simulink model "Sub4"  (R2024a)
settings: Solver=FixedStepDiscrete  StartTime=0.0  StopTime=4.5  FixedStep=75e-6  RelTol=1e-3  EnableMultiTasking=on
undefined symbols (not defined in the file or in its folder): D1, D11, Delta
libraries: spsSeriesRLCBranchLib x41, spsLoadFlowBusLib x29, spsDistributedParametersLineLib x19, spsThreePhaseSeriesRLCLoadLib x15, spsThreePhaseTransformerTwoWindingsLib x13, spsThreePhaseParallelRLCLoadLib x11, spsThreePhaseVIMeasurementLib x11, spsSynchronousMachinepuStandardLib x7, spsExcitationSystemLib x7, spsHydraulicTurbineandGovernorLib x7, spsGenericPowerSystemStabilizerLib x7, spsMultiBandPowerSystemStabilizerLib x7
(part 1 of 5)
settings Model: Creator=The MathWorks, Inc.  LastModifiedBy=dilu2
settings SolverCC: AlgebraicLoopSolver=TrustRegion
settings DataIOCC: SaveFormat=StructureWithTime  SaveOutput=off  SignalLogging=off  DSMLogging=off  SaveTime=off  ReturnWorkspaceOutputs=off
settings OptimizationCC: ExpressionDepthLimit=2147483647  LifeSpan=inf
settings DebuggingCC: UnderspecifiedInitializationDetection=Classic  MergeDetectMultiDrivingBlocksExec=none  SolverPrmCheckMsg=warning  FcnCallInpInsideContextMsg=warning  UnconnectedInputMsg=warning  UnconnectedOutputMsg=warning  UnconnectedLineMsg=warning  StateNameClashWarn=warning  SFUnexpectedBacktrackingDiag=warning  SFNoUnconditionalDefaultTransitionDiag=warning  SFExecutionAtInitializationDiag=none  ArithmeticOperatorsInVariantConditions=warning
settings HardwareCC: ProdBitPerPointer=32  ProdBitPerSizeT=32  ProdBitPerPtrDiffT=32  ProdLargestAtomicFloat=None  ProdIntDivRoundTo=Undefined  ProdEndianess=Unspecified  ProdWordSize=32  ProdHWDeviceType=32-bit Generic
settings ModelReferenceCC: EnableRefExpFcnMdlSchedulingChecks=on  PropagateSignalLabelsOutOfModel=off
settings SFSimCC: SimUseLocalCustomCode=off  CustomCodeUndefinedFunction=UseInterfaceOnly
settings RTWCC: RTWUseLocalCustomCode=off  GPUComputeCapability=3.5
settings CodeAppCC: StateflowObjectComments=on
settings GRTTargetCC: TargetLangStandard=C89/C90 (ANSI)  CombineOutputUpdateFcns=off  GRTInterface=on
settings ConfigComp: CovMetricSettings=dw  CovSaveCumulativeToWorkspaceVar=on  CovSaveSingleToWorkspaceVar=on  CovExternalEMLEnable=off  CovSFcnEnable=off
settings SimscapeCC: SimscapeNormalizeSystem=off

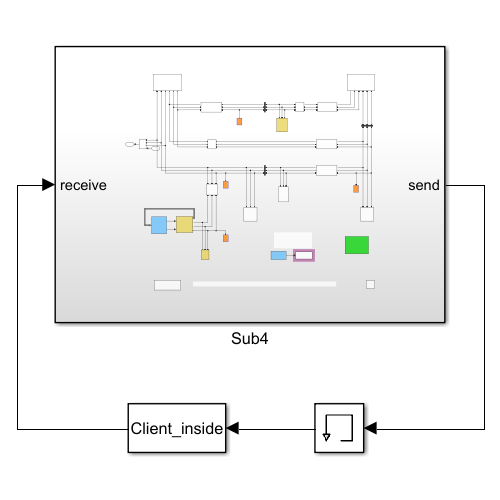
[thumbnail: Simulink's stored preview of the top-level diagram]
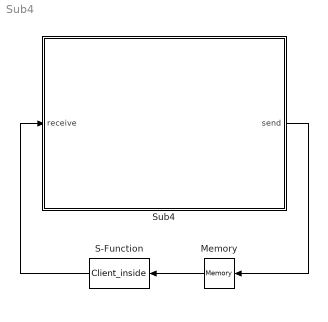
== system Sub4 ==
  Memory : Memory
  S-Function : S-Function  FunctionName=Client_inside  SFunctionDeploymentMode=off  EnableBusSupport=off
  Sub4 : Subsystem
  wires:
  Memory/1 -> S-Function/1
  Sub4/1(send) -> Memory/1
  S-Function/1 -> Sub4/1(receive)

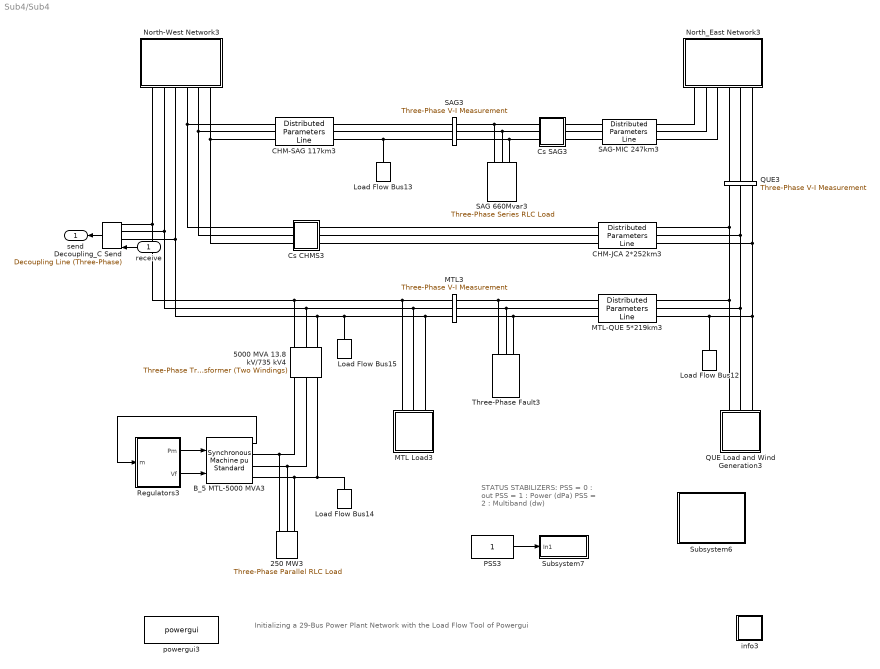
== system Sub4/Sub4 ==
  note: STATUS STABILIZERS:
      | PSS = 0 :  out
      | PSS = 1 :  Power (dPa)
      | PSS = 2 :  Multiband (dw)
  note: Initializing a 29-Bus Power Plant Network with the Load Flow Tool of Powergui
  receive : Inport
  250 MW3 : spsThreePhaseParallelRLCLoadLib/Three-Phase Parallel RLC Load  LConnTagsString=A|B|C  Configuration=Y (grounded)  NominalVoltage=(13800)*1  Vabc=[1e3 1e3 1e3]  Vabcp=[1e3 1e3 1e3]  NominalFrequency=60  UnbalancedPower=off  ActivePower=250000000  InductivePower=0  CapacitivePower=0  Pabc=[10e3 9e3 11e3]  QLabc=[100 90 110]  QCabc=[100 90 110]  Pabcp=[10e3 9e3 11e3]  QLabcp=[100 90 110]  QCabcp=[100 90 110]  Measurements=None  LoadType=constant PQ
  5000 MVA 13.8 kV/735 kV4 : spsThreePhaseTransformerTwoWindingsLib/Three-Phase Transformer (Two Windings)  Winding1Connection=Delta (D1)  Winding2Connection=Yg  CoreType=Three single-phase transformers  SetSaturation=off  Hysteresis=off  DataFile='basic_model'  SetInitialFlux=off  Measurements=None  UNITS=pu  NominalPower=[ 5000e6 60 ]  Winding1="[ 13.8e3 0.002  0.0]"  Winding2=[ 735e3 0.002 0.12]  Rm=500  Lm=500  L0=0.5  Saturation="[ 0,0  ;  0.005,1.2  ;  1.0,1.4 ]"  InitialFluxes=[ 0.8 , -0.8 , 0.7 ]  BreakLoop=off  DiscreteSolver=Trapezoidal iterative  DataType=off  TransfoNumber=0
  B_5 MTL-5000 MVA3 : spsSynchronousMachinepuStandardLib/Synchronous Machine pu Standard  PresetModel=No  MechanicalLoad=Mechanical power Pm  ShowDetailedParameters=on  RotorType=Salient-pole  Units=per unit standard parameters  MeasurementBus=off  NominalParameters="[5000E6  13800   60 ]"  Reactances1=[ 31 32 33 34 35 36 37 ]  Reactances2=[ 1.305, 0.296, 0.252, 0.474, 0.243, 0.18 ]  dAxisTimeConstants=Short-circuit  qAxisTimeConstants=Open-circuit  TimeConstants1=[]  TimeConstants2=[]  TimeConstants3=[]  TimeConstants4=[]  TimeConstants5=[ 1.01, 0.053, 0.1 ]  TimeConstants6=[]  TimeConstants7=[]  TimeConstants8=[]  StatorResistance=2.8544e-3  Mechanical="[ 3.7 0  32]"  PolePairs=32  InitialConditions=[0 -113.876 0.904539 0.904539 0.904539 -42.1129 -162.113 77.8871 1.28555]  SetSaturation=off  Saturation=[0.6404,0.7127,0.8441,0.9214,0.9956,1.082,1.19,1.316,1.457;0.7,0.7698,0.8872,0.9466,0.9969,1.046,1.1,1.151,1.201]  LoadFlowParameters=[1 4000000000 0 0 0]  TsPowergui=0  TsBlock=-1  IterativeModel=Trapezoidal non iterative  IterativeDiscreteModel=Trapezoidal non iterative  BusType=PV  Pref=4500000000  Qref=0  Qmin=-Inf  Qmax=Inf  PLF=0  QLF=0
  CHM-JCA 2*252km3 : spsDistributedParametersLineLib/Distributed Parameters Line  Phases=3  Length=252  Frequency=60  Resistance="[0.01273  0.3864]/2"  Inductance="[0.9337e-3  4.1264e-3]/2"  Capacitance=[12.74e-9 7.751e-9]*2  x1=[-0.0015 2.15568555919851e-08 -52695.4931207272 -817990.56126978;-0.001425 2.15676125923665e-08 -29549.3766895084 -819153.330536763;-0.00135 2.1561128773237e-08 -6379.63893868454 -819661.281164781;-0.001275 2.15374093176625e-08 16795.198597895 -819514.007105874;-0.0012 2.14964731866129e-08 39956.6103096906 -818711.626088671;-0.001125 2.1438353103805e-08 63086.0813185613 -817254.779524281;-0.00105 2.13630955295437e-08 86165.1222792754 -815144.631993557;-0.000975 2.12707606235824e-08 109175.28415961 -812382.870316148;-0.0009 2.11614221970322e-08 132098.172988225 -808971.702202084;-0.000825 2.10351676533583e-08 154915.464558524 -804913.854486961;-0.00075 2.08920979185111e-08 177608.91907674 -800212.570952156;-0.000675 2.07323273602477e-08 200160.395742554 -794871.609731795;-0.0006 2.05559836967078e-08 222551.867250568 -788895.240308557;-0.000525 2.03632078943178e-08 244765.43420106 -782288.240100719;-0.00045 2.01541540551046e-08 266783.339408488 -775055.890643156;-0.000375 1.99289892935087e-08 288587.982096315 -767203.973365366;-0.0003 1.96878936027953e-08 310161.931966798 -758738.764969882;-0.000225 1.94310597111707e-08 331487.943134504 -749667.032414773;-0.00015 1.91586929277182e-08 352548.967912404 -739996.027504242;-7.5e-05 1.88710109782771e-08 373328.170439534 -729733.481091643]  x2=[-0.0015 1.43493457370976e-08 -269861.28631565 -765335.48994974;-0.001425 1.43155296793168e-08 -248116.94439926 -772658.724454069;-0.00135 1.42702700061453e-08 -226174.261593834 -779364.307396144;-0.001275 1.42136028974734e-08 -204050.778544272 -785446.87843556;-0.0012 1.41455736521206e-08 -181764.180424424 -790901.575258095;-0.001125 1.40662366516249e-08 -159332.282799829 -795724.037462569;-0.00105 1.39756553167705e-08 -136773.01738623 -799910.410046481;-0.000975 1.38739020568906e-08 -114104.41771523 -803457.346487641;-0.0009 1.37610582119842e-08 -91344.6047185641 -806362.011419329;-0.000825 1.36372139876944e-08 -68511.7722425057 -808622.082896841;-0.00075 1.35024683831992e-08 -45624.1725039819 -810235.754253618;-0.000675 1.33569291120732e-08 -22700.1015000316 -811201.735545468;-0.0006 1.32007125161829e-08 242.115617734555 -811519.254581725;-0.000525 1.30339434726848e-08 23184.1391919804 -811188.05754253;-0.00045 1.28567552942006e-08 46107.6297200854 -810208.40918173;-0.000375 1.26692896222492e-08 68994.2625144626 -808581.092615234;-0.0003 1.24716963140205e-08 91825.7423510333 -806307.408695007;-0.000225 1.22641333225816e-08 114583.81809415 -803389.174969186;-0.00015 1.20467665706122e-08 137250.297286273 -799828.724229161;-7.5e-05 1.1819769817768e-08 159807.060690745 -795628.902644777]  x3=[-0.0015 5.18178120473788e-11 -353.825063948241 -933.331217283582;-0.001425 5.12281284756022e-11 -327.297425889604 -942.960561677517;-0.00135 5.05974939217388e-11 -300.508151276529 -951.836117826227;-0.001275 4.9926412505402e-11 -273.478655045253 -959.950790745928;-0.0012 4.92154206788081e-11 -246.230544161498 -967.298093691246;-0.001125 4.84650867979448e-11 -218.785600348193 -973.872153340624;-0.00105 4.76760106682359e-11 -191.165762673502 -979.667714491366;-0.000975 4.68488230650662e-11 -163.393110013064 -984.680144260561;-0.0009 4.59841852295494e-11 -135.48984340048 -988.905435788547;-0.000825 4.50827883399416e-11 -107.478268280146 -992.340211441923;-0.00075 4.41453529591247e-11 -79.3807766766213 -994.981725513587;-0.000675 4.31726284585989e-11 -51.2198292947878 -996.827866417607;-0.0006 4.21653924194466e-11 -23.0179375651059 -997.87715837719;-0.000525 4.11244500107463e-11 5.20235435167939 -998.128762604399;-0.00045 4.00506333459326e-11 33.4184875859946 -997.582477970664;-0.000375 3.89448008176175e-11 61.6079065926536 -996.238741167563;-0.0003 3.78078364114041e-11 89.748077181415 -994.098626357737;-0.000225 3.66406489992428e-11 117.816504530469 -991.163844316219;-0.00015 3.54441716128922e-11 145.790751168455 -987.436741062871;-7.5e-05 3.42193606980683e-11 173.648454910629 -982.920295987005]  x4=[-0.0015 3.77673082573545e-11 -3930.11452440301 -10267.8671256384;-0.001425 3.8942548595829e-11 -3638.26562484368 -10374.8700196288;-0.00135 4.00866588567971e-11 -3343.50835141117 -10473.5794012664;-0.001275 4.11987244560214e-11 -3046.07832855995 -10563.9163637817;-0.0012 4.22778564252773e-11 -2746.21331729943 -10645.8086931891;-0.001125 4.33231921229796e-11 -2444.15302513153 -10719.1909260136;-0.00105 4.43338959237659e-11 -2140.13891443214 -10784.0044016209;-0.000975 4.53091598864822e-11 -1834.41400942978 -10840.1973091104;-0.0009 4.62482044000385e-11 -1527.22270193575 -10887.7247287315;-0.000825 4.71502788066187e-11 -1218.81055598109 -10926.5486677923;-0.00075 4.80146620017444e-11 -909.424111516405 -10956.6380910298;-0.000675 4.88406630107148e-11 -599.310687331626 -10977.9689454196;-0.0006 4.96276215409617e-11 -288.718183353157 -10990.5241794029;-0.000525 5.03749085098768e-11 22.1051175235489 -10994.2937565179;-0.00045 5.10819265476911e-11 332.910747907526 -10989.2746634223;-0.000375 5.17481104750028e-11 643.450254533331 -10975.4709123022;-0.0003 5.23729277545734e-11 953.475396870781 -10952.8935376652;-0.000225 5.29558789170297e-11 1262.73834556463 -10921.5605875191;-0.00015 5.34964979601319e-11 1570.99188054559 -10881.4971089448;-7.5e-05 5.39943527212886e-11 1877.98958865422 -10832.7351280741]  x5=0.00142516474882927  V1=ones(3,3)  V2=ones(3,3)  I1=ones(3,3)  I2=ones(3,3)  nHarmo=1  Measurements=None  Decoupling=on  VsMag0=[669271.096488305 669270.65292639 669270.90062483]  VrMag0=[662602.894278686 662603.037872394 662602.72616328]  VsAngle0=[-1.28592943402312 -121.285926872015 118.714104732565]  VrAngle0=[-17.0228975012844 -137.022921456005 102.977079768211]  IsMag0=[819.83811546345 819.831333521039 819.822841412307]  IrMag0=[9030.15416595172 9030.15837069535 9030.16606874901]  IsAngle0=[-18.3607604375278 -138.361719384148 101.639170566751]  IrAngle0=[-18.5448447465977 -138.544772943744 101.455168050312]
      settings: AttributesFormatString=\n  LibrarySourceBlock=sps_lib/Power Grid Elements/Distributed Parameters Line
  CHM-SAG 117km3 : spsDistributedParametersLineLib/Distributed Parameters Line  Phases=3  Length=117  Frequency=60  Resistance="[0.01273  0.3864]"  Inductance="[0.9337e-3  4.1264e-3]"  Capacitance=[12.74e-9 7.751e-9]  x1=[-0.000675 1.98878227916596e-08 120099.384212521 -820048.654169228;-0.0006 1.97251603608904e-08 143234.62761709 -816325.600271039;-0.000525 1.95467299387338e-08 166255.371451905 -811949.988178193;-0.00045 1.93526741597392e-08 189143.213286574 -806925.31568805;-0.000375 1.91431481491271e-08 211879.85693053 -801255.599446916;-0.0003 1.89183193987846e-08 234447.127058726 -794945.371739206;-0.000225 1.86783676333747e-08 256826.983740713 -787999.676864401;-0.00015 1.84234846666673e-08 279001.536861482 -780424.067104709;-7.5e-05 1.81538742482061e-08 300953.060422551 -772224.598286662]  x2=[-0.000675 1.36683940617169e-08 166130.546631601 -803426.098272919;-0.0006 1.35304963284223e-08 188777.466023317 -798408.377649397;-0.000525 1.33817825233862e-08 211273.479597086 -792752.421584839;-0.00045 1.32223715261491e-08 233600.604383858 -786462.751363985;-0.000375 1.3052390767423e-08 255740.992421694 -779544.394852975;-0.0003 1.28719761272257e-08 277676.945023157 -772002.882480148;-0.000225 1.26812718262602e-08 299390.926923368 -763844.242815107;-0.00015 1.24804303106267e-08 320865.580297431 -755074.997749568;-7.5e-05 1.22696121299599e-08 342083.738636013 -745702.157283863]  x3=[-0.000675 1.44875953449933e-11 655.342290943933 -4153.32595111588;-0.0006 1.34518116377455e-11 772.497655199718 -4133.13889809608;-0.000525 1.24052747580941e-11 889.035496649547 -4109.64787708029;-0.00045 1.13488212916082e-11 1004.86265672605 -4082.87166643128;-0.000375 1.02832957510245e-11 1119.88654496969 -4052.83167064216;-0.0003 9.20954990115717e-12 1234.01521304411 -4019.55190322593;-0.000225 8.12844207800969e-12 1347.15742823829 -3983.05896751947;-0.00015 7.04083650263438e-12 1459.22274639654 -3943.38203541722;-7.5e-05 5.94760259028728e-12 1570.12158421818 -3900.55282405163]  x4=[-0.000675 2.92966755964294e-11 -58.1790322608717 -1899.19040567978;-0.0006 2.9950337942892e-11 -4.46495442944831 -1900.07615984023;-0.000525 3.05800584474585e-11 49.2526926182299 -1899.44302219064;-0.00045 3.11853337211928e-11 102.930967817021 -1897.29149885157;-0.000375 3.17656799163019e-11 156.526961575035 -1893.62330971785;-0.0003 3.23206331129171e-11 209.997830074909 -1888.44138708375;-0.000225 3.28497496899441e-11 263.300829522496 -1881.74987329894;-0.00015 3.3352606679687e-11 316.3933503156 -1873.55411745715;-7.5e-05 3.38288021059622e-11 369.232951105443 -1863.86067112021]  x5=0.000661683633385019  V1=ones(3,3)  V2=ones(3,3)  I1=ones(3,3)  I2=ones(3,3)  nHarmo=1  Measurements=None  Decoupling=on  VsMag0=[676709.77841627 676709.532429382 676709.555770597]  VrMag0=[669872.175479969 669872.308250225 669872.011404685]  VsAngle0=[-7.08802978837131 -127.088039531018 112.911983377249]  VrAngle0=[-3.73716141990682 -123.737184181172 116.262817364735]  IsMag0=[3442.59994794247 3442.59576511424 3442.58917191287]  IrMag0=[1555.67453781757 1555.67655932623 1555.68353522262]  IsAngle0=[-6.45330477220923 -126.453471672163 113.546672066868]  IrAngle0=[-17.1748303043271 -137.174490649351 102.825275045855]
      settings: AttributesFormatString=\n  LibrarySourceBlock=sps_lib/Power Grid Elements/Distributed Parameters Line
  Cs CHMS3 : Subsystem  mask{Xc=33/2}
      mask prompts: Xc "Condensator Reactance at  60Hz  (ohm):"
      mask help: Series Compensation
      mask init:
      | Cs=1/Xc/(2*pi*60);
      mask Display: disp('Cs')
  Cs SAG3 : Subsystem  mask{Xc=22}
      mask prompts: Xc "Condensator Reactance at  60Hz  (ohm):"
      mask help: Series Compensation
      mask init:
      | Cs=1/Xc/(2*pi*60);
      mask Display: disp('Cs')
  Decoupling_C Send : spsDecouplingLineThreePhaseLib/Decoupling Line (Three-Phase)  Length=252  Frequency=60  Resistance="[0.01273  0.3864]/2"  Inductance="[0.9337e-3  4.1264e-3]/2"  Capacitance=[12.74e-9 7.751e-9]*2  VsMag0=[645716.873803142 645717.117585011 645717.103800405]  VsAngle0=[95.8608940156725 -144.139117060791 -24.1390927893464]  IhsMag0=[6636.13895490986 6636.14647589719 6636.142035682]  IhsAngle0=[111.871942870307 -128.128050353134 -8.12799750567101]  ShowPorts=on  ConnectorID=T42_4044_2849153755848_S
      settings: LibrarySourceBlock=|
      | sps_lib/Power Grid Elements/Decoupling Line
      | (Three-Phase)
  Load Flow Bus12 : spsLoadFlowBusLib/Load Flow Bus  LConnTagsString=a  Phases=single  Connectors=on one side  ID=QUE7  Vbase=735e3  Vref=1  Vangle=0  VLF=1.023  VLFb=1  VLFc=1  angleLF=-14.99  angleLFb=0  angleLFc=0
      settings: AttributesFormatString=%<ID>\n%<Vbase>V\n%<VLF>pu\n%<angleLF>deg.
  Load Flow Bus13 : spsLoadFlowBusLib/Load Flow Bus  LConnTagsString=a  Phases=single  Connectors=on one side  ID=SAG7  Vbase=735e3  Vref=1  Vangle=0  VLF=1.036  VLFb=1  VLFc=1  angleLF=-0.1653  angleLFb=0  angleLFc=0
      settings: AttributesFormatString=%<ID>\n%<Vbase>V\n%<VLF>pu\n%<angleLF>deg.
  Load Flow Bus14 : spsLoadFlowBusLib/Load Flow Bus  LConnTagsString=a  Phases=single  Connectors=on one side  ID=MTL_13.8  Vbase=13.8e3  Vref=1  Vangle=0  VLF=1  VLFb=1  VLFc=1  angleLF=-47.86  angleLFb=0  angleLFc=0
      settings: AttributesFormatString=%<ID>\n%<Vbase>V\n%<VLF>pu\n%<angleLF>deg.
  Load Flow Bus15 : spsLoadFlowBusLib/Load Flow Bus  LConnTagsString=a  Phases=single  Connectors=on one side  ID=MTL7  Vbase=735e3  Vref=1  Vangle=0  VLF=1.013  VLFb=1  VLFc=1  angleLF=-23.64  angleLFb=0  angleLFc=0
      settings: AttributesFormatString=%<ID>\n%<Vbase>V\n%<VLF>pu\n%<angleLF>deg.
  MTL Load3 : Subsystem
  MTL-QUE 5*219km3 : spsDistributedParametersLineLib/Distributed Parameters Line  Phases=3  Length=219  Frequency=60  Resistance="[0.01273  0.3864]/5"  Inductance="[0.9337e-3  4.1264e-3]/5"  Capacitance=[12.74e-9 7.751e-9]*5  x1=[-0.001275 8.97990123474719e-08 0 0;-0.0012 8.97669453653995e-08 0 0;-0.001125 8.96631200606823e-08 0 0;-0.00105 8.94876194296804e-08 0 0;-0.000975 8.92405837649128e-08 0 0;-0.0009 8.89222105429104e-08 0 0;-0.000825 8.85327542663553e-08 -163872.45963864 -773673.870997357;-0.00075 8.80725262606363e-08 -141934.751428743 -777997.405054978;-0.000675 8.75418944249794e-08 -119883.582750228 -781699.019890759;-0.0006 8.69412829383551e-08 -97736.5809699434 -784775.756490434;-0.000525 8.62711719203961e-08 -75511.450062251 -787225.155357843;-0.00045 8.55320970475971e-08 -53225.9564567427 -789045.258481008;-0.000375 8.47246491251032e-08 -30897.9148360274 -790234.61089734;-0.0003 8.38494736144293e-08 -8545.1738949461 -790792.261856716;-0.000225 8.2907270117488e-08 13814.3979274013 -790717.76558149;-0.00015 8.18987918173386e-08 36162.9267314129 -790011.181622847;-7.5e-05 8.08248448761039e-08 58482.5474451067 -788673.074813191]  x2=[-0.001275 1.42136028974734e-08 0 0;-0.0012 1.41455736521206e-08 0 0;-0.001125 1.40662366516249e-08 0 0;-0.00105 1.39756553167705e-08 0 0;-0.000975 1.38739020568906e-08 0 0;-0.0009 1.37610582119842e-08 0 0;-0.000825 1.36372139876944e-08 -68511.7722425057 -808622.082896841;-0.00075 1.35024683831992e-08 -45624.1725039819 -810235.754253618;-0.000675 1.33569291120732e-08 -22700.1015000316 -811201.735545468;-0.0006 1.32007125161829e-08 242.115617734555 -811519.254581725;-0.000525 1.30339434726848e-08 23184.1391919804 -811188.05754253;-0.00045 1.28567552942006e-08 46107.6297200854 -810208.40918173;-0.000375 1.26692896222492e-08 68994.2625144626 -808581.092615234;-0.0003 1.24716963140205e-08 91825.7423510333 -806307.408695007;-0.000225 1.22641333225816e-08 114583.81809415 -803389.174969186;-0.00015 1.20467665706122e-08 137250.297286273 -799828.724229161;-7.5e-05 1.1819769817768e-08 159807.060690745 -795628.902644777]  x3=[-0.001275 3.56612733394778e-10 0 0;-0.0012 3.31049358806165e-10 0 0;-0.001125 3.05221348425347e-10 0 0;-0.00105 2.79149348768642e-10 0 0;-0.000975 2.52854201393659e-10 0 0;-0.0009 2.26356926238881e-10 0 0;-0.000825 1.99678704820645e-10 -7102.47823834737 -20057.5471743822;-0.00075 1.72840863300962e-10 -6532.60058481158 -20250.3213202489;-0.000675 1.4586485543971e-10 -5957.50087032043 -20426.9076690924;-0.0006 1.18772245444827e-10 -5377.63882078636 -20587.1650604875;-0.000525 9.15846907342113e-11 -4793.4779690596 -20730.9653871275;-0.00045 6.43239246231154e-11 -4205.48528438703 -20858.1936972313;-0.000375 3.70117389508649e-11 -3614.13079912422 -20968.7482864347;-0.0003 9.66996666079572e-12 -3019.88723299863 -21062.5407790905;-0.000225 -1.76795356526667e-11 -2423.22961522482 -21139.4961989151;-0.00015 -4.50149052158343e-11 -1824.63490477324 -21199.5530289235;-7.5e-05 -7.23142905525236e-11 -1224.58160909665 -21242.6632606046]  x4=[-0.001275 2.96404447143572e-10 0 0;-0.0012 3.25528984273917e-10 0 0;-0.001125 3.54393298514994e-10 0 0;-0.00105 3.82974316175637e-10 0 0;-0.000975 4.11249190027634e-10 0 0;-0.0009 4.39195317569445e-10 0 0;-0.000825 4.66790359094306e-10 -1323.85659522578 -8328.03394763841;-0.00075 4.94012255548238e-10 -1087.88942341657 -8362.1315609207;-0.000675 5.20839246163726e-10 -851.052609447551 -8389.5446141781;-0.0006 5.47249885854939e-10 -613.535477044081 -8410.25119383526;-0.000525 5.73223062360603e-10 -375.52789376767 -8424.23474736923;-0.00045 5.98738013120823e-10 -137.22011923875 -8431.48409654126;-0.000375 6.23774341874353e-10 101.197346953951 -8431.99344633255;-0.0003 6.48312034963056e-10 339.533917535869 -8425.76238957667;-0.000225 6.72331477330517e-10 577.599069899151 -8412.79590728505;-0.00015 6.95813468202016e-10 815.202498403518 -8393.10436466524;-7.5e-05 7.18739236433337e-10 1052.15426650368 -8366.70350283512]  x5=0.00123853603172068  V1=ones(3,3)  V2=ones(3,3)  I1=ones(3,3)  I2=ones(3,3)  nHarmo=1  Measurements=None  Decoupling=on  VsMag0=[645717.103800436 645717.117585008 645716.873803144]  VrMag0=[662602.894278686 662603.037872394 662602.72616328]  VsAngle0=[-24.139092789334 -144.139117060794 95.8608940156766]  VrAngle0=[-17.0228975012844 -137.022921456005 102.977079768211]  IsMag0=[17463.0562889063 17463.0593352231 17463.0444100092]  IrMag0=[6920.72764335847 6920.7290374947 6920.73301494311]  IsAngle0=[-31.6792680234199 -151.679318797617 88.3206979336619]  IrAngle0=[-21.2124174849684 -141.212372798418 98.7875948627529]
      settings: AttributesFormatString=\n  LibrarySourceBlock=sps_lib/Power Grid Elements/Distributed Parameters Line
  MTL3 : spsThreePhaseVIMeasurementLib/Three-Phase V-I Measurement  VoltageMeasurement=phase-to-ground  SetLabelV=on  LabelV=Vabc_MTL7_4  Vpu=on  VpuLL=off  CurrentMeasurement=no  SetLabelI=off  LabelI=A1  Ipu=off  Pbase=100e6  Vbase=735e3  OutputType=Magnitude  PhasorSimulation=off  PSBequivalent=0
  North-West Network3 : Subsystem
  North_East Network3 : Subsystem
  PSS3 : Constant
  QUE Load and Wind Generation3 : Subsystem
  QUE3 : spsThreePhaseVIMeasurementLib/Three-Phase V-I Measurement  VoltageMeasurement=no  SetLabelV=on  LabelV=Vabc_QUE7  Vpu=on  VpuLL=off  CurrentMeasurement=no  SetLabelI=off  LabelI=A1  Ipu=off  Pbase=100e6  Vbase=735e3  OutputType=Magnitude  PhasorSimulation=off  PSBequivalent=0
  Regulators3 : Subsystem
  SAG 660Mvar3 : spsThreePhaseSeriesRLCLoadLib/Three-Phase Series RLC Load  LConnTagsString=A|B|C  Configuration=Y (grounded)  NominalVoltage=735e3  Vabc=[1e3 1e3 1e3]  Vabcp=[1e3 1e3 1e3]  NominalFrequency=60  UnbalancedPower=off  ActivePower=2200000  InductivePower=660e6  CapacitivePower=0  Pabc=[10e3 9e3 11e3]  QLabc=[100 90 110]  QCabc=[100 90 110]  Pabcp=[10e3 9e3 11e3]  QLabcp=[100 90 110]  QCabcp=[100 90 110]  Measurements=None  LoadType=constant Z
  SAG-MIC 247km3 : spsDistributedParametersLineLib/Distributed Parameters Line  Phases=3  Length=247  Frequency=60  Resistance="[0.01273  0.3864]/1"  Inductance="[0.9337e-3  4.1264e-3]/1"  Capacitance=[12.74e-9 7.751e-9]*1  x1=[-0.001425 1.51518681270064e-08 -89449.2345901318 -803563.355727012;-0.00135 1.51308920077656e-08 -66696.2840152404 -805770.95443022;-0.001275 1.50978204849643e-08 -43890.0174513944 -807334.432161166;-0.0012 1.50526799954717e-08 -21048.6658791376 -808252.539099673;-0.001125 1.49955066239044e-08 1809.51167456759 -808524.541325103;-0.00105 1.49263460737809e-08 24666.2427323266 -808150.221403037;-0.000975 1.48452536309868e-08 47503.2559730517 -807129.878559095;-0.0009 1.47522941195801e-08 70302.2958377759 -805464.328439734;-0.000825 1.46475418499719e-08 93045.1371228687 -803154.902460235;-0.00075 1.45310805595237e-08 115713.599548984 -800203.446740392;-0.000675 1.44030033456092e-08 138289.562294097 -796612.320628749;-0.0006 1.42634125911935e-08 160754.978479013 -792384.394816571;-0.000525 1.411241988299e-08 183091.889593767 -787523.049043066;-0.00045 1.39501459222593e-08 205282.43985338 -782032.169393661;-0.000375 1.37767204283227e-08 227308.8904715 -775916.145193537;-0.0003 1.35922820348667e-08 249153.63384052 -769179.865498861;-0.000225 1.33969781791208e-08 270799.207606827 -761828.715188551;-0.00015 1.31909649839992e-08 292228.308629939 -753868.57065969;-7.5e-05 1.29744071332979e-08 313423.806814376 -745305.795130019]  x2=[-0.001425 4.7973148933537e-09 11099.4849218348 -821643.782394164;-0.00135 4.75742811271664e-09 34323.407660177 -821001.616626567;-0.001275 4.71373831683737e-09 57519.8927916012 -819703.154728386;-0.0012 4.66628043067023e-09 80670.3974008118 -817749.434670193;-0.001125 4.6150923913233e-09 103756.415328639 -815142.018225911;-0.00105 4.56021511773203e-09 126759.491965578 -811882.989724351;-0.000975 4.50169247794927e-09 149661.239004126 -807974.954383031;-0.0009 4.43957125407784e-09 172443.349138107 -803421.036225608;-0.000825 4.37390110487363e-09 195087.610697259 -798224.875584581;-0.00075 4.3047345260491e-09 217575.92220536 -792390.626191262;-0.000675 4.23212680830911e-09 239890.306850274 -785922.951855348;-0.0006 4.15613599315226e-09 262012.926854336 -778827.022736746;-0.000525 4.07682282647349e-09 283926.097733603 -771108.511212621;-0.00045 3.99425071000473e-09 305612.302434556 -762773.587342989;-0.000375 3.90848565063247e-09 327054.205336969 -753828.913938461;-0.0003 3.81959620763294e-09 348234.666111732 -744281.641234101;-0.000225 3.7276534378668e-09 369136.753422575 -734139.401173629;-0.00015 3.63273083897744e-09 389743.758460713 -723410.301308568;-7.5e-05 3.53490429063805e-09 410039.208301618 -712102.91831719]  x3=[-0.001425 1.52352364734082e-11 -974.267486517483 -4064.81506907934;-0.00135 1.46237071125974e-11 -858.963058340483 -4090.73328748384;-0.001275 1.4000487784071e-11 -742.971988237222 -4113.38143628864;-0.0012 1.33660766798247e-11 -626.386997694417 -4132.74141091012;-0.001125 1.27209809383884e-11 -509.301282969697 -4148.79773528078;-0.00105 1.20657162394275e-11 -391.808440591942 -4161.53757422059;-0.000975 1.14008063915164e-11 -274.002392541647 -4170.95074369723;-0.0009 1.07267829134142e-11 -155.977311171133 -4177.02971896705;-0.000825 1.00441846091762e-11 -37.8275439246008 -4179.76964059022;-0.00075 9.35355713744285e-12 80.3524620817634 -4179.16831831532;-0.000675 8.65545257524804e-12 198.468235559374 -4175.22623283018;-0.0006 7.95042897669744e-12 316.425356566143 -4167.94653537762;-0.000525 7.23904992686851e-12 434.129531984345 -4157.3350452364;-0.00045 6.52188409128923e-12 551.486670897082 -4143.40024506938;-0.000375 5.79950476135553e-12 668.402959803134 -4126.15327414259;-0.0003 5.07248939605101e-12 784.784937610027 -4105.60791942072;-0.000225 4.34141916033498e-12 900.539570345406 -4081.78060454598;-0.00015 3.60687846056811e-12 1015.57432552697 -4054.69037670929;-7.5e-05 2.86945447734696e-12 1129.79724613151 -4024.35889142431]  x4=[-0.001425 1.01505527346392e-11 -279.355223170682 -1839.3774898862;-0.00135 1.08412752682552e-11 -227.24359166425 -1846.54010495214;-0.001275 1.15233314522989e-11 -174.950305107586 -1852.2266241112;-0.0012 1.21961760614925e-11 -122.517165953849 -1856.43250164696;-0.001125 1.28592712341503e-11 -69.986088452223 -1859.15437544527;-0.00105 1.35120869021369e-11 -17.3990651423115 -1860.39006968187;-0.000975 1.41541012145959e-11 35.20186671406 -1860.13859656169;-0.0009 1.47848009551089e-11 87.7746587367869 -1858.40015710849;-0.000825 1.54036819519535e-11 140.277285040317 -1855.17614100417;-0.00075 1.60102494811298e-11 192.6677758285 -1850.46912547788;-0.000675 1.66040186618361e-11 244.904250944602 -1844.28287324581;-0.0006 1.7184514844074e-11 296.944953349659 -1836.62232950334;-0.000525 1.77512739880775e-11 348.748282502419 -1827.49361797194;-0.00045 1.83038430352585e-11 400.272827614174 -1816.90403600391;-0.000375 1.88417802703753e-11 451.477400751914 -1804.86204874907;-0.0003 1.93646556746329e-11 502.321069763328 -1791.37728238777;-0.000225 1.98720512694333e-11 552.763190997344 -1776.46051643593;-0.00015 2.03635614505016e-11 602.763441794037 -1760.123675128;-7.5e-05 2.08387933121192e-11 652.28185271795 -1742.37981788497]  x5=0.00139688767047948  V1=ones(3,3)  V2=ones(3,3)  I1=ones(3,3)  I2=ones(3,3)  nHarmo=1  Measurements=None  Decoupling=on  VsMag0=[660159.37133947 660159.297704423 660159.177083972]  VrMag0=[670930.718084451 670931.402748886 670930.538861588]  VsAngle0=[-5.57176017470454 -125.571775952735 114.428237470918]  VrAngle0=[1.55396261635725 -118.446088813397 121.553886266157]  IsMag0=[3432.79562093234 3432.79304132175 3432.78494377896]  IrMag0=[1527.90652507635 1527.91221755734 1527.91604324796]  IsAngle0=[-12.6984164906756 -132.698597410841 107.301530336567]  IrAngle0=[-7.85604515007248 -127.85575625126 112.143914434317]
      settings: AttributesFormatString=\n  LibrarySourceBlock=sps_lib/Power Grid Elements/Distributed Parameters Line
  SAG3 : spsThreePhaseVIMeasurementLib/Three-Phase V-I Measurement  VoltageMeasurement=no  SetLabelV=on  LabelV=Vabc_SAG7  Vpu=on  VpuLL=off  CurrentMeasurement=no  SetLabelI=off  LabelI=Iabc_SAG7  Ipu=off  Pbase=100e6  Vbase=735e3  OutputType=Magnitude  PhasorSimulation=off  PSBequivalent=0
  Subsystem6 : Subsystem
      mask Display: disp('Display\nWaveforms')
  Subsystem7 : Subsystem
      mask Display: disp('PSS_select')
  Three-Phase Fault3 : spsThreePhaseFaultLib/Three-Phase Fault  InitialStates=0  FaultA=on  FaultB=on  FaultC=on  GroundFault=on  SwitchTimes=[0.2 0.3]  External=off  SwitchStatus=NaN  FaultResistance=0.001  GroundResistance=0.001  SnubberResistance=1e6  SnubberCapacitance=inf  Measurements=None
  info3 : Subsystem
      settings: OpenFcn="showExample(\"simscapeelectricalsps/LoadFlow29BusNetworkExample\")"
      mask Display: disp('?')
  powergui3 : spspowerguiLib/powergui  Priority=1  SimulationMode=Discrete  SampleTime=75e-6  frequency=60  Iterations=50  frequencyindice=60  Pbase=1e+008  ErrMax=0.0001  UnitsV=kV  UnitsW=MW  buscounter=0  FunctionMessages=off  echomessages=off  EnableUseOfTLC=off  CurrentSourceSwitches=off  DisableSnubberDevices=off  DisableRonSwitches=off  DisableVfSwitches=off  DisplayEquations=off  AutomaticDiscreteSolvers=off  SolverType=Tustin/Backward Euler (TBE)  Interpol=off  ExternalGateDelay=off  methode=off  Ts=100  x0status=blocks  SPID=off  SwTol=0  HookPort=off  NonlinearTolerance=1e-4  nMaxIteration=100  ContinueOnMaxIteration=off  RestoreLinks=warning  ResistiveCurrentMeasurement=off  Frange=[0:2:500]  Ylog=off  Xlog=on  ShowGrid=off  save=off  variable=ZData  structure=0  ZoomFFT=off  StartTime=0.0  cycles=1  DisplayStyle=1  fundamental=60  FreqAxis=off  MaxFrequency=1000  frequencyindicesteady=1  RmsSteady=1  display=off
  send : Outport
  wires:
  B_5 MTL-5000 MVA3/1 -> Regulators3/1(m)
  receive/1 -> Decoupling_C Send/1
  PSS3/1 -> Subsystem7/1(In1)
  Regulators3/2(Vf) -> B_5 MTL-5000 MVA3/2
  Decoupling_C Send/1 -> send/1
  Regulators3/1(Pm) -> B_5 MTL-5000 MVA3/1
  connections:
  CHM-JCA 2*252km3/RConn3 -- QUE3/LConn3 -- QUE Load and Wind Generation3/LConn3 -- MTL-QUE 5*219km3/RConn3 -- Load Flow Bus12/LConn1
  SAG3/RConn3 -- SAG 660Mvar3/LConn3 -- Cs SAG3/LConn3
  CHM-JCA 2*252km3/RConn1 -- QUE3/LConn1 -- QUE Load and Wind Generation3/LConn1 -- MTL-QUE 5*219km3/RConn1
  CHM-JCA 2*252km3/RConn2 -- QUE3/LConn2 -- QUE Load and Wind Generation3/LConn2 -- MTL-QUE 5*219km3/RConn2
  SAG3/RConn1 -- SAG 660Mvar3/LConn1 -- Cs SAG3/LConn1
  MTL-QUE 5*219km3/LConn1 -- MTL3/RConn1 -- Three-Phase Fault3/LConn1
  MTL Load3/LConn1 -- MTL3/LConn1 -- North-West Network3/RConn1 -- Decoupling_C Send/LConn3 -- 5000 MVA 13.8 kV/735 kV4/RConn1
  MTL-QUE 5*219km3/LConn2 -- MTL3/RConn2 -- Three-Phase Fault3/LConn2
  SAG-MIC 247km3/RConn1 -- North_East Network3/LConn1
  CHM-SAG 117km3/LConn3 -- North-West Network3/RConn6 -- Cs CHMS3/LConn3
  SAG-MIC 247km3/RConn2 -- North_East Network3/LConn2
  SAG3/LConn1 -- CHM-SAG 117km3/RConn1
  CHM-SAG 117km3/RConn3 -- SAG3/LConn3 -- Load Flow Bus13/LConn1
  SAG3/LConn2 -- CHM-SAG 117km3/RConn2
  QUE3/RConn3 -- North_East Network3/LConn6
  SAG3/RConn2 -- SAG 660Mvar3/LConn2 -- Cs SAG3/LConn2
  250 MW3/LConn2 -- 5000 MVA 13.8 kV/735 kV4/LConn2 -- B_5 MTL-5000 MVA3/RConn2
  Cs CHMS3/RConn1 -- CHM-JCA 2*252km3/LConn1
  MTL-QUE 5*219km3/LConn3 -- MTL3/RConn3 -- Three-Phase Fault3/LConn3
  5000 MVA 13.8 kV/735 kV4/LConn3 -- Load Flow Bus14/LConn1 -- 250 MW3/LConn3 -- B_5 MTL-5000 MVA3/RConn3
  Cs SAG3/RConn1 -- SAG-MIC 247km3/LConn1
  Cs SAG3/RConn3 -- SAG-MIC 247km3/LConn3
  North-West Network3/RConn2 -- MTL3/LConn2 -- MTL Load3/LConn2 -- 5000 MVA 13.8 kV/735 kV4/RConn2 -- Decoupling_C Send/LConn2
  5000 MVA 13.8 kV/735 kV4/RConn3 -- North-West Network3/RConn3 -- Decoupling_C Send/LConn1 -- MTL3/LConn3 -- MTL Load3/LConn3 -- Load Flow Bus15/LConn1
  Cs SAG3/RConn2 -- SAG-MIC 247km3/LConn2
  SAG-MIC 247km3/RConn3 -- North_East Network3/LConn3
  Cs CHMS3/RConn2 -- CHM-JCA 2*252km3/LConn2
  CHM-SAG 117km3/LConn2 -- North-West Network3/RConn5 -- Cs CHMS3/LConn2
  QUE3/RConn2 -- North_East Network3/LConn5
  QUE3/RConn1 -- North_East Network3/LConn4
  250 MW3/LConn1 -- 5000 MVA 13.8 kV/735 kV4/LConn1 -- B_5 MTL-5000 MVA3/RConn1
  Cs CHMS3/RConn3 -- CHM-JCA 2*252km3/LConn3
  CHM-SAG 117km3/LConn1 -- North-West Network3/RConn4 -- Cs CHMS3/LConn1

== system Sub4/Sub4/Cs CHMS3 ==
  note: B
  Ca : spsSeriesRLCBranchLib/Series RLC Branch  LConnTagsString=__new0  RConnTagsString=__new0  BranchType=C  Resistance=1.0  Inductance=1.0  SetiL0=off  InitialCurrent=0  Capacitance=Cs  Setx0=off  InitialVoltage=0  Measurements=None
  Cb : spsSeriesRLCBranchLib/Series RLC Branch  LConnTagsString=__new0  RConnTagsString=__new0  BranchType=C  Resistance=1.0  Inductance=1.0  SetiL0=off  InitialCurrent=0  Capacitance=Cs  Setx0=off  InitialVoltage=0  Measurements=None
  Cc : spsSeriesRLCBranchLib/Series RLC Branch  LConnTagsString=__new0  RConnTagsString=__new0  BranchType=C  Resistance=1.0  Inductance=1.0  SetiL0=off  InitialCurrent=0  Capacitance=Cs  Setx0=off  InitialVoltage=0  Measurements=None
  A : PMIOPort  Side=Left
  B : PMIOPort  Port=2  Side=Left
  C : PMIOPort  Port=3  Side=Left
  "A " : PMIOPort  Port=4  Side=Right
  "B " : PMIOPort  Port=5  Side=Right
  "C " : PMIOPort  Port=6  Side=Right
  connections:
  Cc/RConn1 -- "C "/RConn1
  C/RConn1 -- Cc/LConn1
  Cb/RConn1 -- "B "/RConn1
  B/RConn1 -- Cb/LConn1
  Ca/RConn1 -- "A "/RConn1
  A/RConn1 -- Ca/LConn1

== system Sub4/Sub4/Cs SAG3 ==
  note: B
  Ca : spsSeriesRLCBranchLib/Series RLC Branch  LConnTagsString=__new0  RConnTagsString=__new0  BranchType=C  Resistance=1.0  Inductance=1.0  SetiL0=off  InitialCurrent=0  Capacitance=Cs  Setx0=off  InitialVoltage=0  Measurements=None
  Cb : spsSeriesRLCBranchLib/Series RLC Branch  LConnTagsString=__new0  RConnTagsString=__new0  BranchType=C  Resistance=1.0  Inductance=1.0  SetiL0=off  InitialCurrent=0  Capacitance=Cs  Setx0=off  InitialVoltage=0  Measurements=None
  Cc : spsSeriesRLCBranchLib/Series RLC Branch  LConnTagsString=__new0  RConnTagsString=__new0  BranchType=C  Resistance=1.0  Inductance=1.0  SetiL0=off  InitialCurrent=0  Capacitance=Cs  Setx0=off  InitialVoltage=0  Measurements=None
  A : PMIOPort  Side=Left
  B : PMIOPort  Port=2  Side=Left
  C : PMIOPort  Port=3  Side=Left
  "A " : PMIOPort  Port=4  Side=Right
  "B " : PMIOPort  Port=5  Side=Right
  "C " : PMIOPort  Port=6  Side=Right
  connections:
  A/RConn1 -- Ca/LConn1
  Ca/RConn1 -- "A "/RConn1
  B/RConn1 -- Cb/LConn1
  Cb/RConn1 -- "B "/RConn1
  C/RConn1 -- Cc/LConn1
  Cc/RConn1 -- "C "/RConn1

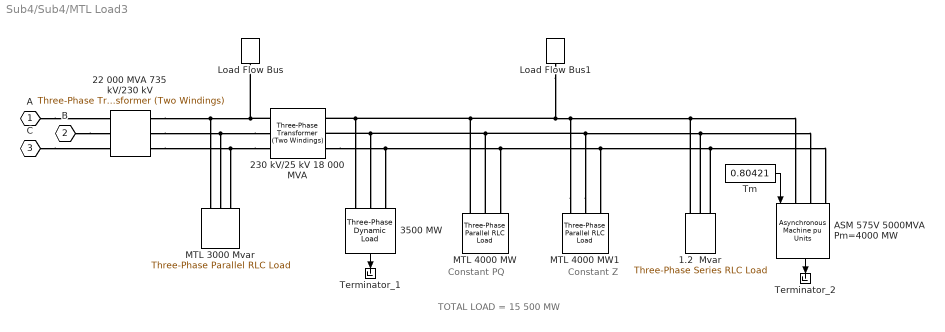
== system Sub4/Sub4/MTL Load3 ==
  note: Constant PQ
  note: Constant Z
  note: TOTAL LOAD = 15 500 MW
  1.2  Mvar : spsThreePhaseSeriesRLCLoadLib/Three-Phase Series RLC Load  LConnTagsString=A|B|C  Configuration=Y (grounded)  NominalVoltage=25e3  Vabc=[1e3 1e3 1e3]  Vabcp=[1e3 1e3 1e3]  NominalFrequency=60  UnbalancedPower=off  ActivePower=2000e6/50  InductivePower=0  CapacitivePower=2000e6  Pabc=[10e3 9e3 11e3]  QLabc=[100 90 110]  QCabc=[100 90 110]  Pabcp=[10e3 9e3 11e3]  QLabcp=[100 90 110]  QCabcp=[100 90 110]  Measurements=None  LoadType=constant Z
  22 000 MVA 735 kV/230 kV : spsThreePhaseTransformerTwoWindingsLib/Three-Phase Transformer (Two Windings)  Winding1Connection=Yg  Winding2Connection=Delta (D1)  CoreType=Three single-phase transformers  SetSaturation=off  Hysteresis=off  DataFile='basic_model'  SetInitialFlux=off  Measurements=None  UNITS=pu  NominalPower=[ 22000e6 60 ]  Winding1="[ 735e3 0.002  0.12]"  Winding2=[230e3 0.002 0]  Rm=500  Lm=500  L0=0.5  Saturation="[ 0,0  ;  0.005,1.2  ;  1.0,1.4 ]"  InitialFluxes=[ 0.8 , -0.8 , 0.7 ]  BreakLoop=off  DiscreteSolver=Trapezoidal iterative  DataType=off  TransfoNumber=0
  230 kV/25 kV 18 000 MVA : spsThreePhaseTransformerTwoWindingsLib/Three-Phase Transformer (Two Windings)  Winding1Connection=Yg  Winding2Connection=Delta (D1)  CoreType=Three single-phase transformers  SetSaturation=off  Hysteresis=off  DataFile='basic_model'  SetInitialFlux=off  Measurements=None  UNITS=pu  NominalPower=[18000e6 60 ]  Winding1="[ 230e3  0.08/30   0.08 ]"  Winding2="[ 25e3  0.08/30  0.08]"  Rm=500  Lm=500  L0=0.5  Saturation="[ 0,0  ;  0.005,1.2  ;  1.0,1.4 ]"  InitialFluxes=[ 0.8 , -0.8 , 0.7 ]  BreakLoop=off  DiscreteSolver=Trapezoidal iterative  DataType=off  TransfoNumber=0
  3500 MW : spsThreePhaseDynamicLoadLib/Three-Phase Dynamic Load  NominalVoltage=[ 25e3 60 ]  ActiveReactivePowers=[3.5e+09 4.44089e-08]  PositiveSequence=[0.991615 -96.3945]  ExternalControl=off  NpNq="[1.5  2.5]"  TimeConstants="[0  0  0  0]"  MinimumVoltage=0.7  Tfilter=1e-4  LoadFlowParameters=[4,0,0,0,0]
      settings: LibrarySourceBlock=|
      | sps_lib/Passives/Three-Phase
      | Dynamic Load
  ASM 575V 5000MVA Pm=4000 MW : spsAsynchronousMachinepuUnitsLib/Asynchronous Machine pu Units  RotorType=Squirrel-cage  PresetModel=No  MechanicalLoad=Torque Tm  ShowDetailedParameters=on  ReferenceFrame=Rotor  Units=pu  MeasurementBus=off  NominalParameters="[5000e6 25e3  60]"  VoltageRatio=1  Stator=[0.01117 0.04832]  Rotor=[0.006 0.04832]  Cage1=[0.01909 0.0397]  Cage2=[0.01909 0.0397]  Lm=2.424  Mechanical="[1  0   2]"  PolePairs=2  InitialConditions=[0.00523668 0 0.941796 0.941796 0.941796 -125.733 -245.733 -5.73298]  SimulateSaturation=off  Saturation="[0.212,0.4201,0.8125,1.0979,1.4799,2.2457,3.2586,4.5763,6.4763 ;   0.5,0.7,0.9,1,1.1,1.2 ,1.3,1.4,1.5]"  LoadFlowParameters=0  TsPowergui=0  TsBlock=-1  IterativeModel=Trapezoidal non iterative  IterativeDiscreteModel=Trapezoidal non iterative  Pmec=4000000000
      settings: LibrarySourceBlock=|
      | sps_lib/Electrical Machines/Asynchronous Machine
      | pu Units
  Load Flow Bus : spsLoadFlowBusLib/Load Flow Bus  LConnTagsString=a  Phases=single  Connectors=on one side  ID=MTL2  Vbase=230e3  Vref=1  Vangle=0  VLF=1.009  VLFb=1  VLFc=1  angleLF=-58.45  angleLFb=0  angleLFc=0
      settings: AttributesFormatString=%<ID>\n%<Vbase>V\n%<VLF>pu\n%<angleLF>deg.
  Load Flow Bus1 : spsLoadFlowBusLib/Load Flow Bus  LConnTagsString=a  Phases=single  Connectors=on one side  ID=MTL_25  Vbase=25e3  Vref=1  Vangle=0  VLF=0.9916  VLFb=1  VLFc=1  angleLF=-96.39  angleLFb=0  angleLFc=0
      settings: AttributesFormatString=%<ID>\n%<Vbase>V\n%<VLF>pu\n%<angleLF>deg.
  MTL 3000 Mvar : spsThreePhaseParallelRLCLoadLib/Three-Phase Parallel RLC Load  LConnTagsString=A|B|C  Configuration=Y (grounded)  NominalVoltage=230e3  Vabc=[1e3 1e3 1e3]  Vabcp=[1e3 1e3 1e3]  NominalFrequency=60  UnbalancedPower=off  ActivePower=0  InductivePower=0  CapacitivePower=3000e6  Pabc=[10e3 9e3 11e3]  QLabc=[100 90 110]  QCabc=[100 90 110]  Pabcp=[10e3 9e3 11e3]  QLabcp=[100 90 110]  QCabcp=[100 90 110]  Measurements=None  LoadType=constant Z
  MTL 4000 MW : spsThreePhaseParallelRLCLoadLib/Three-Phase Parallel RLC Load  LConnTagsString=A|B|C  Configuration=Y (grounded)  NominalVoltage=(25000)*0.991615  Vabc=[1e3 1e3 1e3]  Vabcp=[1e3 1e3 1e3]  NominalFrequency=60  UnbalancedPower=off  ActivePower=4000000000  InductivePower=0  CapacitivePower=0  Pabc=[10e3 9e3 11e3]  QLabc=[100 90 110]  QCabc=[100 90 110]  Pabcp=[10e3 9e3 11e3]  QLabcp=[100 90 110]  QCabcp=[100 90 110]  Measurements=None  LoadType=constant PQ
  MTL 4000 MW1 : spsThreePhaseParallelRLCLoadLib/Three-Phase Parallel RLC Load  LConnTagsString=A|B|C  Configuration=Y (grounded)  NominalVoltage=25e3  Vabc=[1e3 1e3 1e3]  Vabcp=[1e3 1e3 1e3]  NominalFrequency=60  UnbalancedPower=off  ActivePower=4000000000  InductivePower=0  CapacitivePower=0  Pabc=[10e3 9e3 11e3]  QLabc=[100 90 110]  QCabc=[100 90 110]  Pabcp=[10e3 9e3 11e3]  QLabcp=[100 90 110]  QCabcp=[100 90 110]  Measurements=None  LoadType=constant Z
  Terminator_1 : Terminator
  Terminator_2 : Terminator
  Tm : Constant  Value=0.80421
  A : PMIOPort  Side=Left
  B : PMIOPort  Port=2  Side=Left
  C : PMIOPort  Port=3  Side=Left
  wires:
  Tm/1 -> ASM 575V 5000MVA Pm=4000 MW/1
  3500 MW/1 -> Terminator_1/1
  ASM 575V 5000MVA Pm=4000 MW/1 -> Terminator_2/1
  connections:
  A/RConn1 -- 22 000 MVA 735 kV/230 kV/LConn1
  B/RConn1 -- 22 000 MVA 735 kV/230 kV/LConn2
  C/RConn1 -- 22 000 MVA 735 kV/230 kV/LConn3
  230 kV/25 kV 18 000 MVA/LConn1 -- Load Flow Bus/LConn1 -- 22 000 MVA 735 kV/230 kV/RConn1 -- MTL 3000 Mvar/LConn1
  230 kV/25 kV 18 000 MVA/LConn2 -- 22 000 MVA 735 kV/230 kV/RConn2 -- MTL 3000 Mvar/LConn2
  230 kV/25 kV 18 000 MVA/LConn3 -- 22 000 MVA 735 kV/230 kV/RConn3 -- MTL 3000 Mvar/LConn3
  MTL 4000 MW1/LConn1 -- Load Flow Bus1/LConn1 -- MTL 4000 MW/LConn1 -- 230 kV/25 kV 18 000 MVA/RConn1 -- 3500 MW/LConn1 -- ASM 575V 5000MVA Pm=4000 MW/LConn1 -- 1.2  Mvar/LConn1
  MTL 4000 MW1/LConn2 -- MTL 4000 MW/LConn2 -- 230 kV/25 kV 18 000 MVA/RConn2 -- 3500 MW/LConn2 -- ASM 575V 5000MVA Pm=4000 MW/LConn2 -- 1.2  Mvar/LConn2
  230 kV/25 kV 18 000 MVA/RConn3 -- ASM 575V 5000MVA Pm=4000 MW/LConn3 -- 1.2  Mvar/LConn3 -- MTL 4000 MW1/LConn3 -- MTL 4000 MW/LConn3 -- 3500 MW/LConn3
